simulink model "arduino_lab_R2016a"  (R2016a)
settings: Solver=VariableStepAuto  StartTime=0.0  StopTime=500  RelTol=1e-3
StartFcn:
  | clear all
libraries: simulink x1, realtime_pacer_lib x1
settings Model: Creator=johnh  LastModifiedBy=johnh

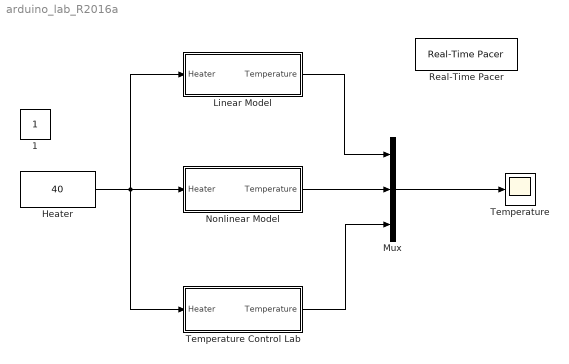
== system arduino_lab_R2016a ==
  Heater : simulink/Math Operations/Slider Gain  gain=40  low=0  high=100
  Linear Model : Subsystem
  Mux : Mux  Inputs=3
  Nonlinear Model : Subsystem
  Real-Time Pacer : realtime_pacer_lib/Real-Time Pacer  simTimePerRealTime=1
  Temperature : Scope
  Temperature Control Lab : Subsystem
  1 : Constant  IOType=siggen
  wires:
  Mux/1 -> Temperature/1
  Linear Model/1(Temperature) -> Mux/1
  Nonlinear Model/1(Temperature) -> Mux/2
  Temperature Control Lab/1(Temperature) -> Mux/3
  Heater/1 -> Linear Model/1(Heater), Temperature Control Lab/1(Heater), Nonlinear Model/1(Heater)

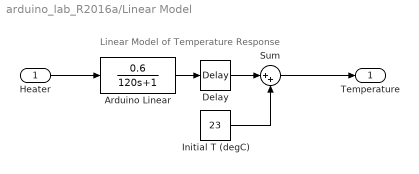
== system arduino_lab_R2016a/Linear Model ==
  note: Linear Model of Temperature Response
  Heater : Inport
  Arduino Linear : TransferFcn  Numerator=[0.6]  Denominator=[120 1]
  Delay : TransportDelay  DelayTime=3
  Initial T (degC) : Constant  Value=23
  Sum : Sum  Inputs=|++
  Temperature : Outport
  wires:
  Arduino Linear/1 -> Delay/1
  Delay/1 -> Sum/1
  Initial T (degC)/1 -> Sum/2
  Sum/1 -> Temperature/1
  Heater/1 -> Arduino Linear/1

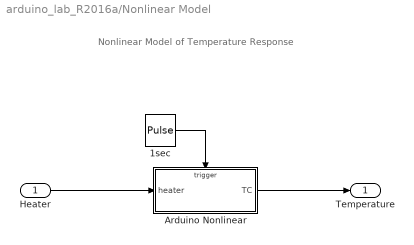
== system arduino_lab_R2016a/Nonlinear Model ==
  note: Nonlinear Model of Temperature Response
  Heater : Inport
  1sec : DiscretePulseGenerator  PulseType=Time based  Period=1  PulseWidth=50
  Arduino Nonlinear : Subsystem  TreatAsAtomicUnit=on
  Temperature : Outport
  wires:
  1sec/1 -> Arduino Nonlinear/Trigger
  Arduino Nonlinear/1(TC) -> Temperature/1
  Heater/1 -> Arduino Nonlinear/1(heater)

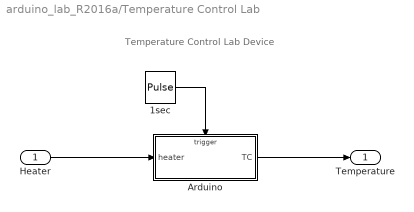
== system arduino_lab_R2016a/Temperature Control Lab ==
  note: Temperature Control Lab Device
  Heater : Inport
  1sec : DiscretePulseGenerator  PulseType=Time based  Period=1  PulseWidth=50
  Arduino : Subsystem  TreatAsAtomicUnit=on
  Temperature : Outport
  wires:
  1sec/1 -> Arduino/Trigger
  Arduino/1(TC) -> Temperature/1
  Heater/1 -> Arduino/1(heater)

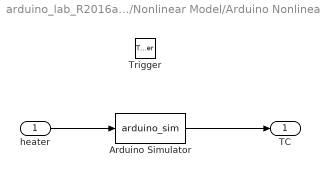
== system arduino_lab_R2016a/Nonlinear Model/Arduino Nonlinear ==
  heater : Inport
  Trigger : TriggerPort  VariantControl=Variant
  Arduino Simulator : MATLABFcn  MATLABFcn=arduino_sim
  TC : Outport  InitialOutput=23
  wires:
  heater/1 -> Arduino Simulator/1
  Arduino Simulator/1 -> TC/1

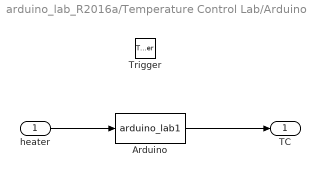
== system arduino_lab_R2016a/Temperature Control Lab/Arduino ==
  heater : Inport  LatchByDelayingOutsideSignal=on
  Trigger : TriggerPort  VariantControl=Variant
  Arduino : MATLABFcn  MATLABFcn=arduino_lab1
  TC : Outport  InitialOutput=23
  wires:
  heater/1 -> Arduino/1
  Arduino/1 -> TC/1
